simulink model "test1"  (Simulink 8.1)
settings: Solver=VariableStepDiscrete  StartTime=0.0  StopTime=1000  RelTol=1e-3
undefined symbols (not defined in the file or in its folder): fdesignblkfcn, gcbh
libraries: simulink x2, commchan3 x1, commdigbbndpm3 x1, commrandsrc2 x1
settings Model: Creator=Gaurav  LastModifiedBy=Gaurav
settings OptimizationCC: InitFltsAndDblsToZero=on
settings DebuggingCC: StrictBusMsg=Warning

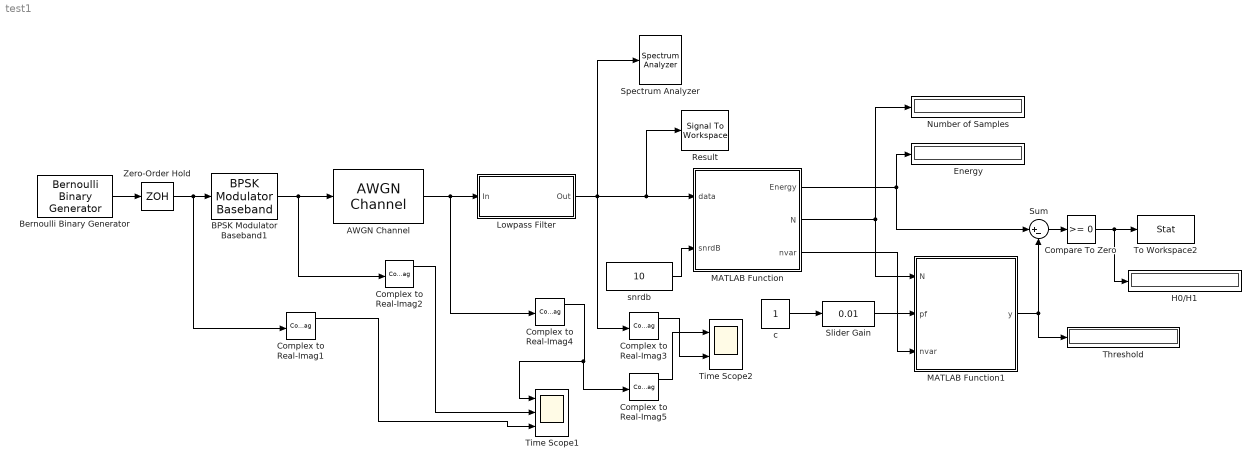
== system test1 ==
  AWGN Channel : commchan3/AWGN Channel  InputProcessing=Columns as channels (frame based)  seed=67  noiseMode="Signal to noise ratio  (SNR)"  EbNodB=2  EsNodB=10  SNRdB=8  bitsPerSym=1  Ps=1  Tsym=1/3200  variance=1
  BPSK Modulator Baseband1 : commdigbbndpm3/BPSK Modulator Baseband  Ph=0  outDtype=double  outWordLen=16  outUDDataType=sfix(16)  outFracLenMode=Best precision  outFracLen=15
  Bernoulli Binary Generator : commrandsrc2/Bernoulli Binary Generator  P=0.5  seed=61  Ts=1  frameBased=off  sampPerFrame=100  orient=off  outDataType=double
  Compare To Zero : simulink/Logic and Bit Operations/Compare To Zero  relop=>=  OutDataTypeStr=boolean
  Complex to Real-Imag{1..5} (5 alike) : ComplexToRealImag
  Energy : Display
  H0/H1 : Display
  Lowpass Filter : Subsystem  DialogController=fdesignblkfcn  DialogControllerArgs=DataTag2  InitFcn=fdesignblkfcn(gcbh, {'InitFcn'});  mask(Lowpass Filter){}
      mask help: Design a lowpass filter
      settings: CopyFcn=fdesignblkfcn(gcbh, {'CopyFcn'});
      mask Help: helpview(mapfilelocation('dspblks'), 'dsplowpassfilter')
      mask Display: disp('Lowpass')
  MATLAB Function : MATLAB Function  TreatAsAtomicUnit=on
  MATLAB Function1 : MATLAB Function  TreatAsAtomicUnit=on
  Number of Samples : Display
  Result : SignalToWorkspace  VariableName=data
      settings: CopyFcn=dspblkcopystw(gcbh);
  Slider Gain : simulink/Math Operations/Slider Gain  low=0.01  gain=0.01  high=1
  Spectrum Analyzer : SpectrumAnalyzer
      settings: CopyFcn=scopeextensions.ScopeBlock.callback(gcbh, 'onBlockCopy', gcbh);  DeleteFcn=scopeextensions.ScopeBlock.callback(gcbh, 'onBlockDelete');  PreSaveFcn=scopeextensions.ScopeBlock.callback(gcbh, 'onModelSave');  NameChangeFcn=scopeextensions.ScopeBlock.callback(gcbh, 'onBlockRename');  CloseFcn=scopeextensions.ScopeBlock.callback(gcbh, 'onBlockClose');  PreDeleteFcn=scopeextensions.ScopeBlock.callback(gcbh, 'onBlockPreDelete');
  Sum : Sum  Inputs=|+-
  Threshold : Display
  Time Scope1 : Scope  NumInputPorts=3
      settings: YMin=-2~-2~-5  YMax=2~2~5  DataFormat=Structure
  Time Scope2 : Scope  NumInputPorts=2
      settings: TimeRange=350  YMin=-3.001326621702043~-5  YMax=3.552804503074786~5  DataFormat=Structure
  To Workspace2 : ToWorkspace  VariableName=Stat  SampleTime=-1
  Zero-Order Hold : ZeroOrderHold  SampleTime=1/32
  c : Constant
  snrdb : Constant  Value=10
  wires:
  Bernoulli Binary Generator/1 -> Zero-Order Hold/1
  Complex to Real-Imag1/1 -> Time Scope1/3
  Complex to Real-Imag2/1 -> Time Scope1/2
  Complex to Real-Imag5/1 -> Time Scope2/1
  Complex to Real-Imag3/1 -> Time Scope2/2
  MATLAB Function/1(Energy) -> Energy/1, Sum/1
  MATLAB Function/2(N) -> Number of Samples/1, MATLAB Function1/1(N)
  c/1 -> Slider Gain/1
  MATLAB Function1/1(y) -> Threshold/1, Sum/2
  Sum/1 -> Compare To Zero/1
  Compare To Zero/1 -> H0/H1/1, To Workspace2/1
  Slider Gain/1 -> MATLAB Function1/2(pf)
  snrdb/1 -> MATLAB Function/2(snrdB)
  MATLAB Function/3(nvar) -> MATLAB Function1/3(nvar)
  Zero-Order Hold/1 -> Complex to Real-Imag1/1, BPSK Modulator Baseband1/1
  BPSK Modulator Baseband1/1 -> Complex to Real-Imag2/1, AWGN Channel/1
  AWGN Channel/1 -> Complex to Real-Imag4/1, Lowpass Filter/1(In)
  Complex to Real-Imag4/1 -> Complex to Real-Imag5/1, Time Scope1/1
  Lowpass Filter/1(Out) -> Spectrum Analyzer/1, Complex to Real-Imag3/1, MATLAB Function/1(data), Result/1

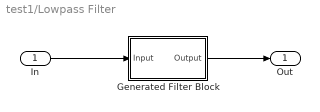
== system test1/Lowpass Filter ==
  In : Inport
  Generated Filter Block : Subsystem  Tag=FilterWizardSubSystem
      settings: ErrorFcn=dspFilterRealizedInBasicElemsAlgLoopErrFcnCallback
  Out : Outport
  wires:
  In/1 -> Generated Filter Block/1(Input)
  Generated Filter Block/1(Output) -> Out/1

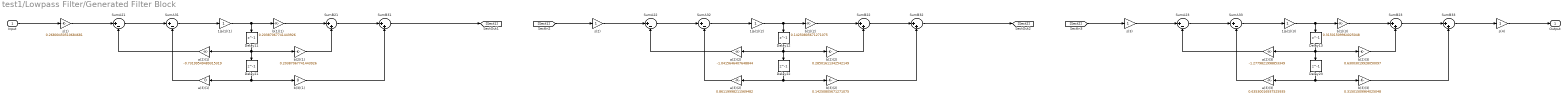
== system test1/Lowpass Filter/Generated Filter Block ==
  Input : Inport
  1|a(1)(1) : Gain  ParamDataTypeStr=double  RndMeth=Nearest  SaturateOnIntegerOverflow=on  OutDataTypeStr=Inherit: Same as input
  1|a(1)(2) : Gain  ParamDataTypeStr=double  RndMeth=Nearest  SaturateOnIntegerOverflow=on  OutDataTypeStr=Inherit: Same as input
  1|a(1)(3) : Gain  ParamDataTypeStr=double  RndMeth=Nearest  SaturateOnIntegerOverflow=on  OutDataTypeStr=Inherit: Same as input
  Delay{11..13,21..23} (6 alike) : Delay  DelayLength=1  InitialCondition=0  InputProcessing=Inherited
  SumA{21..23,31..33} (6 alike) : Sum  Inputs=|+-  RndMeth=Nearest  SaturateOnIntegerOverflow=on  OutDataTypeStr=Inherit: Same as first input
  SumB{21..23,31..33} (6 alike) : Sum  Inputs=|++  RndMeth=Nearest  SaturateOnIntegerOverflow=on  OutDataTypeStr=Inherit: Same as first input
  a(2)(1) : Gain  Gain=-0.73199549489315319  ParamDataTypeStr=double  RndMeth=Nearest  SaturateOnIntegerOverflow=on  OutDataTypeStr=Inherit: Same as input
  a(2)(2) : Gain  Gain=-1.0415646407648844  ParamDataTypeStr=double  RndMeth=Nearest  SaturateOnIntegerOverflow=on  OutDataTypeStr=Inherit: Same as input
  a(2)(3) : Gain  Gain=-1.2779821998853349  ParamDataTypeStr=double  RndMeth=Nearest  SaturateOnIntegerOverflow=on  OutDataTypeStr=Inherit: Same as input
  a(3)(1) : Gain  Gain=0  ParamDataTypeStr=double  RndMeth=Nearest  SaturateOnIntegerOverflow=on  OutDataTypeStr=Inherit: Same as input
  a(3)(2) : Gain  Gain=0.86119998211569482  ParamDataTypeStr=double  RndMeth=Nearest  SaturateOnIntegerOverflow=on  OutDataTypeStr=Inherit: Same as input
  a(3)(3) : Gain  Gain=0.63530016937525935  ParamDataTypeStr=double  RndMeth=Nearest  SaturateOnIntegerOverflow=on  OutDataTypeStr=Inherit: Same as input
  b(1)(1) : Gain  Gain=0.20387067741443926  ParamDataTypeStr=double  RndMeth=Nearest  SaturateOnIntegerOverflow=on  OutDataTypeStr=Inherit: Same as input
  b(1)(2) : Gain  Gain=0.14250805671271075  ParamDataTypeStr=double  RndMeth=Nearest  SaturateOnIntegerOverflow=on  OutDataTypeStr=Inherit: Same as input
  b(1)(3) : Gain  Gain=0.31501509964025048  ParamDataTypeStr=double  RndMeth=Nearest  SaturateOnIntegerOverflow=on  OutDataTypeStr=Inherit: Same as input
  b(2)(1) : Gain  Gain=0.20387067741443926  ParamDataTypeStr=double  RndMeth=Nearest  SaturateOnIntegerOverflow=on  OutDataTypeStr=Inherit: Same as input
  b(2)(2) : Gain  Gain=0.28501611342542149  ParamDataTypeStr=double  RndMeth=Nearest  SaturateOnIntegerOverflow=on  OutDataTypeStr=Inherit: Same as input
  b(2)(3) : Gain  Gain=0.63003019928050097  ParamDataTypeStr=double  RndMeth=Nearest  SaturateOnIntegerOverflow=on  OutDataTypeStr=Inherit: Same as input
  b(3)(1) : Gain  Gain=0  ParamDataTypeStr=double  RndMeth=Nearest  SaturateOnIntegerOverflow=on  OutDataTypeStr=Inherit: Same as input
  b(3)(2) : Gain  Gain=0.14250805671271075  ParamDataTypeStr=double  RndMeth=Nearest  SaturateOnIntegerOverflow=on  OutDataTypeStr=Inherit: Same as input
  b(3)(3) : Gain  Gain=0.31501509964025048  ParamDataTypeStr=double  RndMeth=Nearest  SaturateOnIntegerOverflow=on  OutDataTypeStr=Inherit: Same as input
  s(1) : Gain  Gain=0.26800450510684681  ParamDataTypeStr=double  RndMeth=Nearest  SaturateOnIntegerOverflow=on  OutDataTypeStr=Inherit: Same as input
  s(2) : Gain  ParamDataTypeStr=double  RndMeth=Nearest  SaturateOnIntegerOverflow=on  OutDataTypeStr=Inherit: Same as input
  s(3) : Gain  ParamDataTypeStr=double  RndMeth=Nearest  SaturateOnIntegerOverflow=on  OutDataTypeStr=Inherit: Same as input
  s(4) : Gain  ParamDataTypeStr=double  RndMeth=Nearest  SaturateOnIntegerOverflow=on  OutDataTypeStr=Inherit: Same as input
  Output : Outport
  wires:
  Input/1 -> s(1)/1
  s(1)/1 -> SumA21/1
  SumA21/1 -> SumA31/1
  SumA31/1 -> 1|a(1)(1)/1
  1|a(1)(1)/1 -> b(1)(1)/1, Delay11/1
  b(1)(1)/1 -> SumB21/1
  SumB21/1 -> SumB31/1
  SumB31/1 -> [Sect1]
  a(2)(1)/1 -> SumA21/2
  Delay11/1 -> a(2)(1)/1, b(2)(1)/1, Delay21/1
  b(2)(1)/1 -> SumB21/2
  a(3)(1)/1 -> SumA31/2
  Delay21/1 -> a(3)(1)/1, b(3)(1)/1
  b(3)(1)/1 -> SumB31/2
  [Sect1] -> s(2)/1
  s(2)/1 -> SumA22/1
  SumA22/1 -> SumA32/1
  SumA32/1 -> 1|a(1)(2)/1
  1|a(1)(2)/1 -> b(1)(2)/1, Delay12/1
  b(1)(2)/1 -> SumB22/1
  SumB22/1 -> SumB32/1
  SumB32/1 -> [Sect2]
  a(2)(2)/1 -> SumA22/2
  Delay12/1 -> a(2)(2)/1, b(2)(2)/1, Delay22/1
  b(2)(2)/1 -> SumB22/2
  a(3)(2)/1 -> SumA32/2
  Delay22/1 -> a(3)(2)/1, b(3)(2)/1
  b(3)(2)/1 -> SumB32/2
  [Sect2] -> s(3)/1
  s(3)/1 -> SumA23/1
  SumA23/1 -> SumA33/1
  SumA33/1 -> 1|a(1)(3)/1
  1|a(1)(3)/1 -> b(1)(3)/1, Delay13/1
  b(1)(3)/1 -> SumB23/1
  SumB23/1 -> SumB33/1
  SumB33/1 -> s(4)/1
  a(2)(3)/1 -> SumA23/2
  Delay13/1 -> a(2)(3)/1, b(2)(3)/1, Delay23/1
  b(2)(3)/1 -> SumB23/2
  a(3)(3)/1 -> SumA33/2
  Delay23/1 -> a(3)(3)/1, b(3)(3)/1
  b(3)(3)/1 -> SumB33/2
  s(4)/1 -> Output/1

== matlab function MATLAB Function ==
  data: data input double; Energy output double; N output double; snrdB input double; nvar output double
function [Energy,N,nvar]= Energy_estimation(data,snrdB)
[m,n]=size(data);
Energy=sum(abs(data).^2);
snr = 10^(snrdB/20);
nvar = 1/snr;
N=m;
% end

== matlab function MATLAB Function1 ==
  data: N input double; pf input double; nvar input double; y output double
% function y = threshold(N,Pfa,noise_power)
% % coder.extrinsic('qfuncinv');
% % coder.extrinsic('sqrt');
% % [m,n]=size(Pfa);
% % t=double(ones(m,n));
% % t=(qfuncinv(Pfa)./712);
% % y=t+1;
% % 
function y = Threshold(N,pf,nvar)
    coder.extrinsic('qfuncinv');
    t=double(zeros(1,1));
    t=qfuncinv(pf);
    thresh=double(zeros(1,1));
    thresh = sqrt(2*N*nvar^4)*t+N*nvar^2;
y=thresh;
